simulink model "computed_torque_controller"  (R2016b)
settings: Solver=FixedStepAuto  StartTime=0.0  StopTime=20  FixedStep=0.3  RelTol=1e-3
undefined symbols (not defined in the file or in its folder): sigbuilder_block
libraries: simulink x4
settings Model: SimulationMode=rapid-accelerator  Creator=jocol  LastModifiedBy=jocol

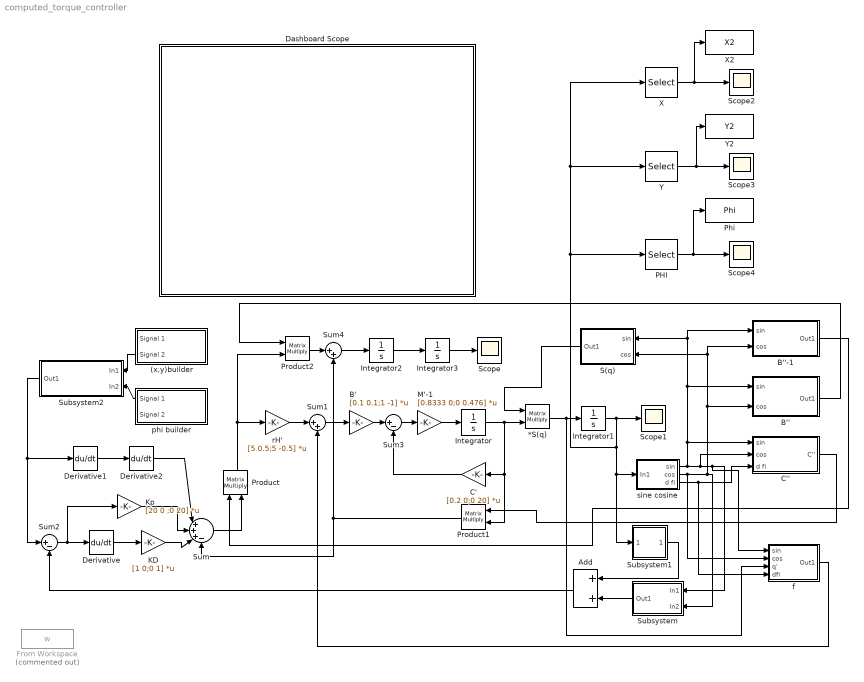
== system computed_torque_controller ==
  (x,y)builder : Subsystem  Tag=STV Subsys  LoadFcn=sigbuilder_block('load');  StartFcn=sigbuilder_block('start');  StopFcn=sigbuilder_block('stop');  ClipboardFcn=sigbuilder_block('clipboard');  mask(Sigbuilder block){tuvar=[0:10]}
      mask help: Simulink:masks:SigbuilderBlock_MD
      mask init:
      | if ~strcmp(get_param(bdroot(gcbh),'SimulationStatus'),'stopped') tuvar = sigbuilder_block('maskInit'); end
      settings: CopyFcn=sigbuilder_block('copy');  DeleteFcn=sigbuilder_block('delete');  ModelCloseFcn=sigbuilder_block('modelClose');  PreSaveFcn=sigbuilder_block('preSave');  PauseFcn=sigbuilder_block('pause');  ContinueFcn=sigbuilder_block('continue');  NameChangeFcn=sigbuilder_block('namechange');  OpenFcn=sigbuilder_block('open',[534 124.8 550.8 385.2 ]);  CloseFcn=sigbuilder_block('close');
      mask Display: plot(0, 0, 100, 100,[2, 2, 32, 32, 2], [68, 8, 8, 68, 68],[32, 2], [38, 38], [32, 19, 2],[53, 60, 44], [32, 17, 17, 2],[16, 16, 31, 31]);txt = getActiveGroup(gcbh);text(2, 100, txt,'verticalAlignment', 'top');
  *S(q) : Product  Multiplication=Matrix(*)
  Add : Sum
  B' : Gain  Gain=[0.1 0.1;1 -1]  Multiplication=Matrix(K*u)
  B'' : Subsystem
  B''-1 : Subsystem
  C' : Gain  Gain=[0.2 0;0 20]  Multiplication=Matrix(K*u) (u vector)
  C'' : Subsystem
  Dashboard Scope : Subsystem  DialogController=hmiCreateDDGDialog  IsWebBlock=on  mask(MWDashboardBlock){webBlockId=2148f017-9aaa-4a70-a443-0d1812a898a8, webBlockType=sdiscope, ShowInitialText=on, HMISrcModelName=computed_torque_controller}
      mask prompts: webBlockId "WebBlock Id"; webBlockType "WebBlock Type"; HMISrcModelName "Source Model"
      mask help: SimulinkHMI:dialogs:HMIScopeDialogDesc
      mask Help: helpview([docroot '/mapfiles/simulink.map'], 'hmi_scope')
      mask Display:
      | if strcmp(get_param(bdroot(gcb),'BlockDiagramType'), 'library')
      |     image([(matlabroot) '/toolbox/simulink/hmi/icons/DashboardScope.png']);
      | end
  Derivative : Derivative
  Derivative1 : Derivative
  Derivative2 : Derivative
  From Workspace : FromWorkspace  Commented=on  VariableName=w
  Integrator : Integrator  UpperSaturationLimit=10
  Integrator1 : Integrator  InitialCondition=[-7;-7;-pi]  UpperSaturationLimit=10
  Integrator2 : Integrator
  Integrator3 : Integrator
  KD : Gain  Gain=[1 0;0 1]  Multiplication=Matrix(K*u)
  Kp : Gain  Gain=[20 0 ;0 20]  Multiplication=Matrix(K*u)
  M'-1 : Gain  Gain=[0.8333 0;0 0.476]  Multiplication=Matrix(K*u)
  PHI : Selector  InputPortWidth=3  IndexOptions=Index vector (dialog)  Indices=3  OutputSizes=1
  Phi : ToWorkspace  VariableName=Phi  SampleTime=-1
  Product : Product  Multiplication=Matrix(*)
  Product1 : Product  Multiplication=Matrix(*)
  Product2 : Product  Multiplication=Matrix(*)
  S(q) : Subsystem
  Scope{,1..4} (5 alike) : Scope
  Subsystem : Subsystem
  Subsystem1 : Subsystem
  Subsystem2 : Subsystem
  Sum : Sum  Inputs=|+++-
  Sum1 : Sum  Inputs=|++
  Sum2 : Sum  Inputs=|+-
  Sum3 : Sum  Inputs=|+-
  Sum4 : Sum  Inputs=|++
  X : Selector  InputPortWidth=3  IndexOptions=Index vector (dialog)  Indices=1  OutputSizes=1
  X2 : ToWorkspace  VariableName=X2  SampleTime=-1
  Y : Selector  InputPortWidth=3  IndexOptions=Index vector (dialog)  Indices=2  OutputSizes=1
  Y2 : ToWorkspace  VariableName=Y2  SampleTime=-1
  f : Subsystem
  phi builder : Subsystem  Tag=STV Subsys  LoadFcn=sigbuilder_block('load');  StartFcn=sigbuilder_block('start');  StopFcn=sigbuilder_block('stop');  ClipboardFcn=sigbuilder_block('clipboard');  mask(Sigbuilder block){tuvar=[0:10]}
      mask help: Simulink:masks:SigbuilderBlock_MD
      mask init:
      | if ~strcmp(get_param(bdroot(gcbh),'SimulationStatus'),'stopped') tuvar = sigbuilder_block('maskInit'); end
      settings: CopyFcn=sigbuilder_block('copy');  DeleteFcn=sigbuilder_block('delete');  ModelCloseFcn=sigbuilder_block('modelClose');  PreSaveFcn=sigbuilder_block('preSave');  PauseFcn=sigbuilder_block('pause');  ContinueFcn=sigbuilder_block('continue');  NameChangeFcn=sigbuilder_block('namechange');  OpenFcn=sigbuilder_block('open',[343.2 19.2 550.8 400.2 ]);  CloseFcn=sigbuilder_block('close');
      mask Display: plot(0, 0, 100, 100,[2, 2, 32, 32, 2], [68, 8, 8, 68, 68],[32, 2], [38, 38], [32, 19, 2],[53, 60, 44], [32, 17, 17, 2],[16, 16, 31, 31]);txt = getActiveGroup(gcbh);text(2, 100, txt,'verticalAlignment', 'top');
  rH' : Gain  Gain=[5 0.5;5 -0.5]  Multiplication=Matrix(K*u)
  sine cosine : Subsystem
  wires:
  Derivative/1 -> KD/1
  Kp/1 -> Sum/2
  Product/1 -> Product2/2, rH'/1
  rH'/1 -> Sum1/1
  Sum1/1 -> B'/1
  Sum2/1 -> Kp/1, Derivative/1
  Sum3/1 -> M'-1/1
  M'-1/1 -> Integrator/1
  C'/1 -> Sum3/2
  *S(q)/1 -> f/3(q'), Integrator1/1
  Integrator1/1 -> PHI/1, X/1, Y/1, sine cosine/1(In1), Subsystem1/1(In1), Scope1/1
  sine cosine/1(sin) -> S(q)/1(sin), B''-1/1(sin), B''/1(sin), C''/1(sin), C''/2(cos), f/1(sin), Subsystem/1(In1)
  sine cosine/2(cos) -> f/2(cos), S(q)/2(cos), B''-1/2(cos), B''/2(cos), Subsystem/2(In2)
  Subsystem/1(Out1) -> Add/2
  B'/1 -> Sum3/1
  sine cosine/3(d fi) -> f/4(dfi), C''/3(d fi)
  C''/1(C'') -> Product1/1
  Product1/1 -> Sum/4, Sum4/2
  f/1(Out1) -> Sum1/2
  B''-1/1(Out1) -> Product/1
  B''/1(Out1) -> Product2/1
  Product2/1 -> Sum4/1
  Sum4/1 -> Integrator2/1
  Integrator2/1 -> Integrator3/1
  Integrator3/1 -> Scope/1
  S(q)/1(Out1) -> *S(q)/1
  Subsystem1/1(Out1) -> Add/1
  Sum/1 -> Product/2
  Integrator/1 -> Product1/2, C'/1, *S(q)/2
  KD/1 -> Sum/3
  Add/1 -> Sum2/2
  Derivative1/1 -> Derivative2/1
  Derivative2/1 -> Sum/1
  PHI/1 -> Phi/1, Scope4/1
  Y/1 -> Y2/1, Scope3/1
  X/1 -> X2/1, Scope2/1
  (x,y)builder/2(Signal 2) -> Subsystem2/1(In1)
  phi builder/1(Signal 1) -> Subsystem2/2(In2)
  Subsystem2/1(Out1) -> Derivative1/1, Sum2/1

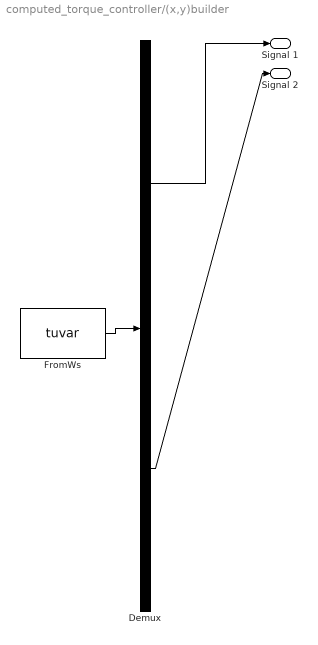
== system computed_torque_controller/(x,y)builder ==
  Demux : Demux  Tag=STV Demux  Outputs=2
  FromWs : FromWorkspace  Tag=STV FromWs  VariableName=tuvar  SampleTime=0
      SigBuilderData=|
      | common.afterFinalStr = 'Extrapolate'
      | common.sampleTime = 0
      | dataSet.timeRange = [0 10]
      | dataSet.name = 'Group 1'
      | sbobj.Groups.Name = 'Group 1'
      | sbobj.Groups.Signals(1).Name = 'Signal 1'
      | sbobj.Groups.Signals(1).XData = [0 8 10]
      | sbobj.Groups.Signals(1).YData = [0 0 0]
      | sbobj.Groups.Signals(2).Name = 'Signal 2'
      | sbobj.Groups.Signals(2).XData = [0 2 9 10]
      | sbobj.Groups.Signals(2).YData = [1 0.9 0 0]
  Signal 1 : Outport  Tag=STV Outport
  Signal 2 : Outport  Tag=STV Outport  Port=2
  wires:
  Demux/1 -> Signal 1/1
  FromWs/1 -> Demux/1
  Demux/2 -> Signal 2/1

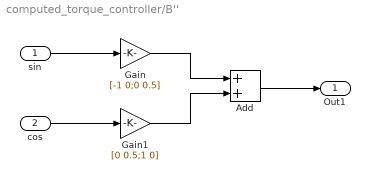
== system computed_torque_controller/B'' ==
  sin : Inport
  cos : Inport  Port=2
  Add : Sum
  Gain : Gain  Gain=[-1 0;0 0.5]
  Gain1 : Gain  Gain=[0 0.5;1 0]
  Out1 : Outport
  wires:
  Gain/1 -> Add/1
  Gain1/1 -> Add/2
  sin/1 -> Gain/1
  cos/1 -> Gain1/1
  Add/1 -> Out1/1

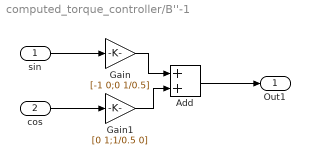
== system computed_torque_controller/B''-1 ==
  sin : Inport
  cos : Inport  Port=2
  Add : Sum
  Gain : Gain  Gain=[-1 0;0 1/0.5]
  Gain1 : Gain  Gain=[0 1;1/0.5 0]
  Out1 : Outport
  wires:
  sin/1 -> Gain/1
  cos/1 -> Gain1/1
  Gain/1 -> Add/1
  Gain1/1 -> Add/2
  Add/1 -> Out1/1

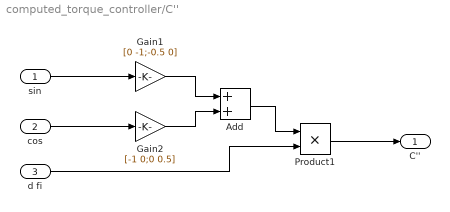
== system computed_torque_controller/C'' ==
  sin : Inport
  cos : Inport  Port=2
  d fi : Inport  Port=3
  Add : Sum
  Gain1 : Gain  Gain=[0 -1;-0.5 0]
  Gain2 : Gain  Gain=[-1 0;0 0.5]
  Product1 : Product
  C'' : Outport
  wires:
  sin/1 -> Gain1/1
  cos/1 -> Gain2/1
  Gain1/1 -> Add/1
  Gain2/1 -> Add/2
  Add/1 -> Product1/1
  d fi/1 -> Product1/2
  Product1/1 -> C''/1

== system computed_torque_controller/Dashboard Scope ==

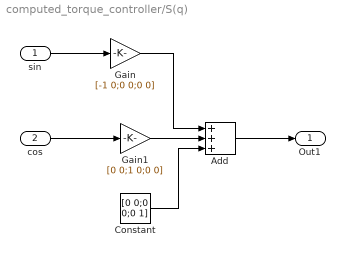
== system computed_torque_controller/S(q) ==
  sin : Inport
  cos : Inport  Port=2
  Add : Sum  Inputs=+++
  Constant : Constant  Value=[0 0;0 0;0 1]
  Gain : Gain  Gain=[-1 0;0 0;0 0]
  Gain1 : Gain  Gain=[0 0;1 0;0 0]
  Out1 : Outport
  wires:
  sin/1 -> Gain/1
  cos/1 -> Gain1/1
  Gain/1 -> Add/1
  Gain1/1 -> Add/2
  Constant/1 -> Add/3
  Add/1 -> Out1/1

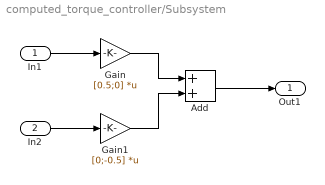
== system computed_torque_controller/Subsystem ==
  In1 : Inport
  In2 : Inport  Port=2
  Add : Sum
  Gain : Gain  Gain=[0.5;0]  Multiplication=Matrix(K*u)
  Gain1 : Gain  Gain=[0;-0.5]  Multiplication=Matrix(K*u)
  Out1 : Outport
  wires:
  In1/1 -> Gain/1
  In2/1 -> Gain1/1
  Gain/1 -> Add/1
  Gain1/1 -> Add/2
  Add/1 -> Out1/1

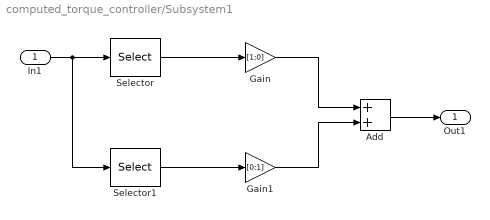
== system computed_torque_controller/Subsystem1 ==
  In1 : Inport
  Add : Sum
  Gain : Gain  Gain=[1;0]
  Gain1 : Gain  Gain=[0;1]
  Selector : Selector  InputPortWidth=3  IndexOptions=Index vector (dialog)  Indices=1  OutputSizes=1
  Selector1 : Selector  InputPortWidth=3  IndexOptions=Index vector (dialog)  Indices=2  OutputSizes=1
  Out1 : Outport
  wires:
  Gain/1 -> Add/1
  Selector/1 -> Gain/1
  In1/1 -> Selector1/1, Selector/1
  Selector1/1 -> Gain1/1
  Gain1/1 -> Add/2
  Add/1 -> Out1/1

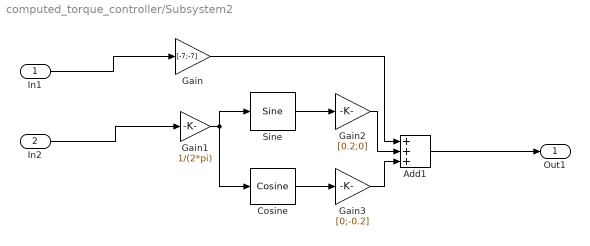
== system computed_torque_controller/Subsystem2 ==
  In1 : Inport
  In2 : Inport  Port=2
  Add1 : Sum  Inputs=+++
  Cosine : simulink/Lookup Tables/Cosine  Formula=cos(2*pi*u)  NumDataPoints=(2^5)+1  OutputWordLength=16  InternalRulePriority=Speed
  Gain : Gain  Gain=[-7;-7]
  Gain1 : Gain  Gain=1/(2*pi)
  Gain2 : Gain  Gain=[0.2;0]
  Gain3 : Gain  Gain=[0;-0.2]
  Sine : simulink/Lookup Tables/Sine  Formula=sin(2*pi*u)  NumDataPoints=(2^5)+1  OutputWordLength=16  InternalRulePriority=Speed
  Out1 : Outport
  wires:
  Gain1/1 -> Sine/1, Cosine/1
  Sine/1 -> Gain2/1
  Cosine/1 -> Gain3/1
  Gain/1 -> Add1/1
  Gain2/1 -> Add1/2
  Gain3/1 -> Add1/3
  In1/1 -> Gain/1
  In2/1 -> Gain1/1
  Add1/1 -> Out1/1

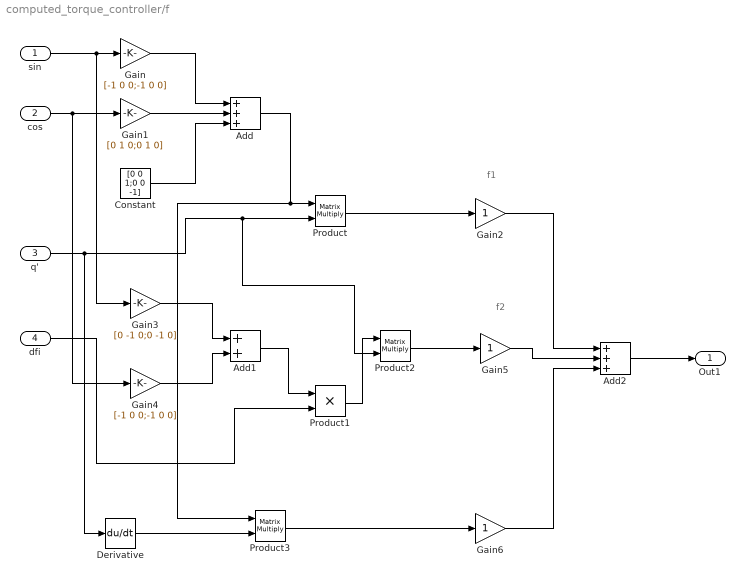
== system computed_torque_controller/f ==
  note: f2
  note: f1
  sin : Inport
  cos : Inport  Port=2
  q' : Inport  Port=3
  dfi : Inport  Port=4
  Add : Sum  Inputs=+++
  Add1 : Sum
  Add2 : Sum  Inputs=+++
  Constant : Constant  Value=[0 0 1;0 0 -1]
  Derivative : Derivative
  Gain : Gain  Gain=[-1 0 0;-1 0 0]
  Gain1 : Gain  Gain=[0 1 0;0 1 0]
  Gain2 : Gain
  Gain3 : Gain  Gain=[0 -1 0;0 -1 0]
  Gain4 : Gain  Gain=[-1 0 0;-1 0 0]
  Gain5 : Gain
  Gain6 : Gain
  Product : Product  Multiplication=Matrix(*)
  Product1 : Product
  Product2 : Product  Multiplication=Matrix(*)
  Product3 : Product  Multiplication=Matrix(*)
  Out1 : Outport
  wires:
  sin/1 -> Gain3/1, Gain/1
  cos/1 -> Gain4/1, Gain1/1
  Gain/1 -> Add/1
  Gain1/1 -> Add/2
  Constant/1 -> Add/3
  Add/1 -> Product3/1, Product/1
  q'/1 -> Derivative/1, Product2/2, Product/2
  Product/1 -> Gain2/1
  Gain3/1 -> Add1/1
  Gain4/1 -> Add1/2
  Add1/1 -> Product1/1
  dfi/1 -> Product1/2
  Product1/1 -> Product2/1
  Product2/1 -> Gain5/1
  Derivative/1 -> Product3/2
  Product3/1 -> Gain6/1
  Gain2/1 -> Add2/1
  Gain5/1 -> Add2/2
  Gain6/1 -> Add2/3
  Add2/1 -> Out1/1

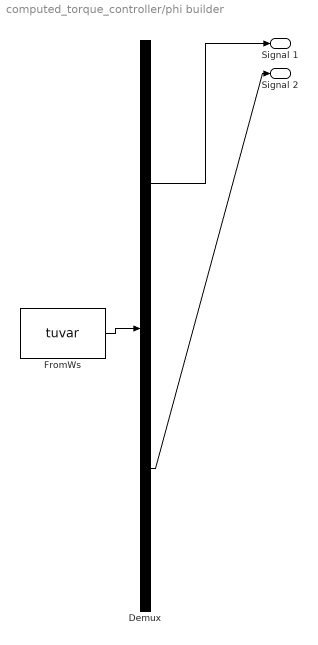
== system computed_torque_controller/phi builder ==
  Demux : Demux  Tag=STV Demux  Outputs=2
  FromWs : FromWorkspace  Tag=STV FromWs  VariableName=tuvar  SampleTime=0
      SigBuilderData=|
      | common.afterFinalStr = 'Extrapolate'
      | common.sampleTime = 0
      | dataSet.timeRange = [0 10]
      | dataSet.name = 'Group 1'
      | sbobj.Groups.Name = 'Group 1'
      | sbobj.Groups.Signals(1).Name = 'Signal 1'
      | sbobj.Groups.Signals(1).XData = [0 2 10]
      | sbobj.Groups.Signals(1).YData = [-3.14159265359 0 0]
      | sbobj.Groups.Signals(2).Name = 'Signal 2'
      | sbobj.Groups.Signals(2).XData = [0 10]
      | sbobj.Groups.Signals(2).YData = [0 0]
  Signal 1 : Outport  Tag=STV Outport
  Signal 2 : Outport  Tag=STV Outport  Port=2
  wires:
  Demux/1 -> Signal 1/1
  FromWs/1 -> Demux/1
  Demux/2 -> Signal 2/1

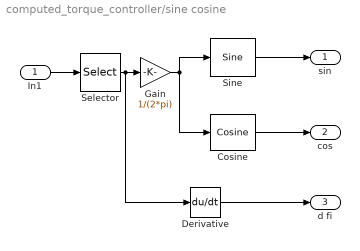
== system computed_torque_controller/sine cosine ==
  In1 : Inport
  Cosine : simulink/Lookup Tables/Cosine  Formula=cos(2*pi*u)  NumDataPoints=(2^5)+1  OutputWordLength=16  InternalRulePriority=Speed
  Derivative : Derivative
  Gain : Gain  Gain=1/(2*pi)
  Selector : Selector  InputPortWidth=3  IndexOptions=Index vector (dialog)  Indices=3  OutputSizes=1
  Sine : simulink/Lookup Tables/Sine  Formula=sin(2*pi*u)  NumDataPoints=(2^5)+1  OutputWordLength=16  InternalRulePriority=Speed
  sin : Outport
  cos : Outport  Port=2
  d fi : Outport  Port=3
  wires:
  Selector/1 -> Derivative/1, Gain/1
  Gain/1 -> Sine/1, Cosine/1
  In1/1 -> Selector/1
  Sine/1 -> sin/1
  Cosine/1 -> cos/1
  Derivative/1 -> d fi/1
